simulink model "a11"  (R2024b)
settings: Solver=VariableStepAuto  StartTime=0.0  StopTime=1  RelTol=1e-3
settings Model: Creator=86195  LastModifiedBy=86195

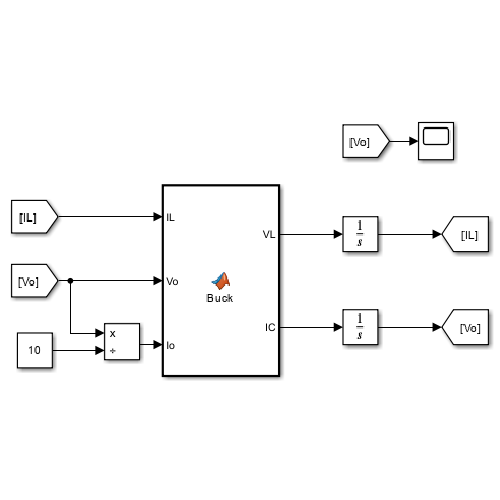
[thumbnail: Simulink's stored preview of the top-level diagram]
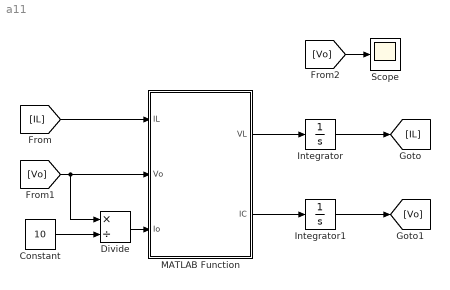
== system a11 ==
  Constant : Constant  Value=10
  Divide : Product  Inputs=*/
  Integrator : Integrator
  Integrator1 : Integrator
  MATLAB Function : MATLAB Function  TreatAsAtomicUnit=on
  Scope : Scope
  wires:
  MATLAB Function/2(IC) -> Integrator1/1
  MATLAB Function/1(VL) -> Integrator/1
  Integrator/1 -> [IL]
  [IL] -> MATLAB Function/1(IL)
  [Vo] -> Divide/1, MATLAB Function/2(Vo)
  Integrator1/1 -> [Vo]
  Divide/1 -> MATLAB Function/3(Io)
  Constant/1 -> Divide/2
  [Vo] -> Scope/1

== matlab function a11/MATLAB Function ==
  data: IL input; VL output; Vo input; Io input; IC output
function [VL,IC]= Buck(IL, Vo, Io)
%% 参 数
Vg = 100;
L = 1e-3;
C = 470e-6;
D = 0.7;
%% 电 感 电 压、 电 容 电 流 公 式
VL = (Vg*D - Vo)/L;
IC = (IL - Io)/C;
